simulink library "reelInOut"  (R2018a)
settings: Solver=VariableStepAuto  StartTime=0.0  StopTime=10.0  RelTol=1e-3
undefined symbols (not defined in the file or in its folder): ctrl, plant
libraries: controllerComponents x9, simulink x6
settings Model: Creator=mitch  LastModifiedBy=mitch

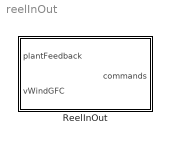
== system reelInOut ==
  ReelInOut : Subsystem  VariantControl=variantOCKReelInOut

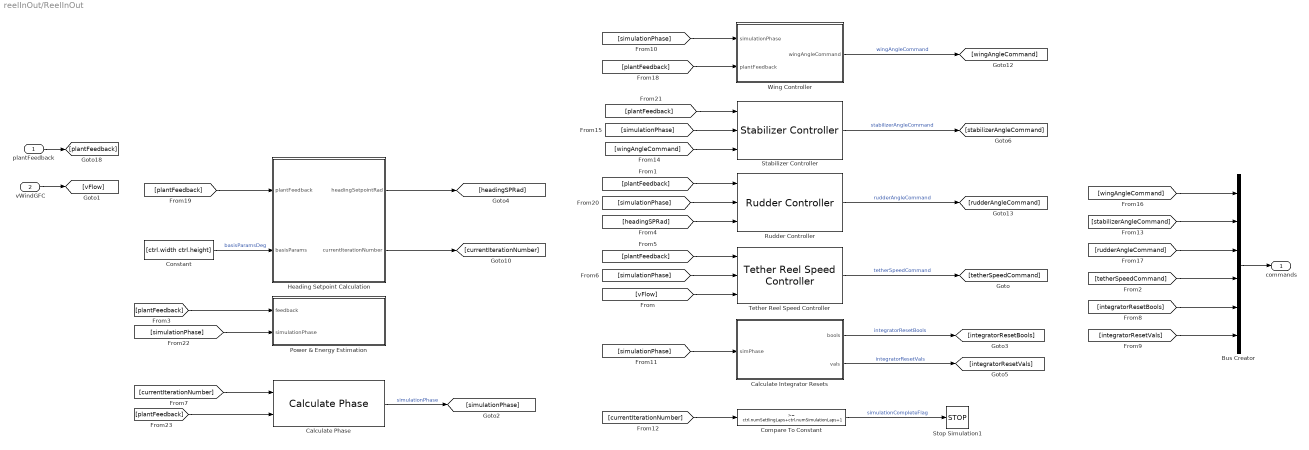
== system reelInOut/ReelInOut ==
  plantFeedback : Inport  OutDataTypeStr=Bus: busPlantFeedback
  vWindGFC : Inport  Port=2
  Bus Creator : BusCreator  Inputs=6  OutDataTypeStr=Bus: busControllerOutput
  Calculate Integrator Resets : Subsystem
  Calculate Phase : controllerComponents/Calculate Phase
  Compare To Constant : simulink/Logic and Bit Operations/Compare To Constant  relop=>=  const=ctrl.numSettlingLaps+ctrl.numSimulationLaps+1  OutDataTypeStr=boolean
  Constant : Constant  Value=[ctrl.width ctrl.height]
  Heading Setpoint Calculation : Subsystem  VariantControl=variantPureCarrotFollowing
  Power & Energy Estimation : Subsystem
  Rudder Controller : controllerComponents/Rudder Controller
  Stabilizer Controller : controllerComponents/Stabilizer Controller
  Stop Simulation1 : Stop
  Tether Reel Speed Controller : controllerComponents/Tether Reel Speed Controller
  Wing Controller : Subsystem
  commands : Outport  OutDataTypeStr=Bus: busControllerOutput
  wires:
  [plantFeedback] -> Calculate Phase/2
  [simulationPhase] -> Power & Energy Estimation/2(simulationPhase)
  [wingAngleCommand] -> Stabilizer Controller/3
  [plantFeedback] -> Stabilizer Controller/1
  [simulationPhase] -> Stabilizer Controller/2
  [simulationPhase] -> Rudder Controller/2
  [headingSPRad] -> Rudder Controller/3
  [plantFeedback] -> Rudder Controller/1
  [stabilizerAngleCommand] -> Bus Creator/2
  Stabilizer Controller/1 -> [stabilizerAngleCommand]  "stabilizerAngleCommand"
  [wingAngleCommand] -> Bus Creator/1
  [rudderAngleCommand] -> Bus Creator/3
  [tetherSpeedCommand] -> Bus Creator/4
  [integratorResetBools] -> Bus Creator/5
  [integratorResetVals] -> Bus Creator/6
  [simulationPhase] -> Tether Reel Speed Controller/2
  [plantFeedback] -> Tether Reel Speed Controller/1
  [vFlow] -> Tether Reel Speed Controller/3
  Calculate Integrator Resets/2(vals) -> [integratorResetVals]  "integratorResetVals"
  Calculate Integrator Resets/1(bools) -> [integratorResetBools]  "integratorResetBools"
  [simulationPhase] -> Calculate Integrator Resets/1(simPhase)
  [simulationPhase] -> Wing Controller/1(simulationPhase)
  Wing Controller/1(wingAngleCommand) -> [wingAngleCommand]  "wingAngleCommand"
  [plantFeedback] -> Wing Controller/2(plantFeedback)
  Calculate Phase/1 -> [simulationPhase]  "simulationPhase"
  [currentIterationNumber] -> Calculate Phase/1
  [plantFeedback] -> Power & Energy Estimation/1(feedback)
  Tether Reel Speed Controller/1 -> [tetherSpeedCommand]  "tetherSpeedCommand"
  Rudder Controller/1 -> [rudderAngleCommand]  "rudderAngleCommand"
  Heading Setpoint Calculation/1(headingSetpointRad) -> [headingSPRad]
  Heading Setpoint Calculation/2(currentIterationNumber) -> [currentIterationNumber]
  Compare To Constant/1 -> Stop Simulation1/1  "simulationCompleteFlag"
  [currentIterationNumber] -> Compare To Constant/1
  Bus Creator/1 -> commands/1
  vWindGFC/1 -> [vFlow]
  plantFeedback/1 -> [plantFeedback]
  Constant/1 -> Heading Setpoint Calculation/2(basisParams)  "basisParamsDeg"
  [plantFeedback] -> Heading Setpoint Calculation/1(plantFeedback)

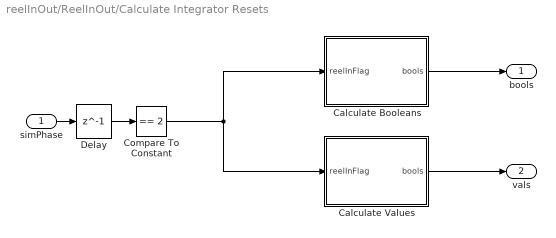
== system reelInOut/ReelInOut/Calculate Integrator Resets ==
  simPhase : Inport
  Calculate Booleans : Subsystem
  Calculate Values : Subsystem
  Compare To Constant : simulink/Logic and Bit Operations/Compare To Constant  relop===  const=2  OutDataTypeStr=boolean
  Delay : Delay  DelayLength=1  InitialCondition=0
  bools : Outport
  vals : Outport  Port=2
  wires:
  Delay/1 -> Compare To Constant/1
  Compare To Constant/1 -> Calculate Values/1(reelInFlag), Calculate Booleans/1(reelInFlag)
  Calculate Values/1(bools) -> vals/1
  Calculate Booleans/1(bools) -> bools/1
  simPhase/1 -> Delay/1

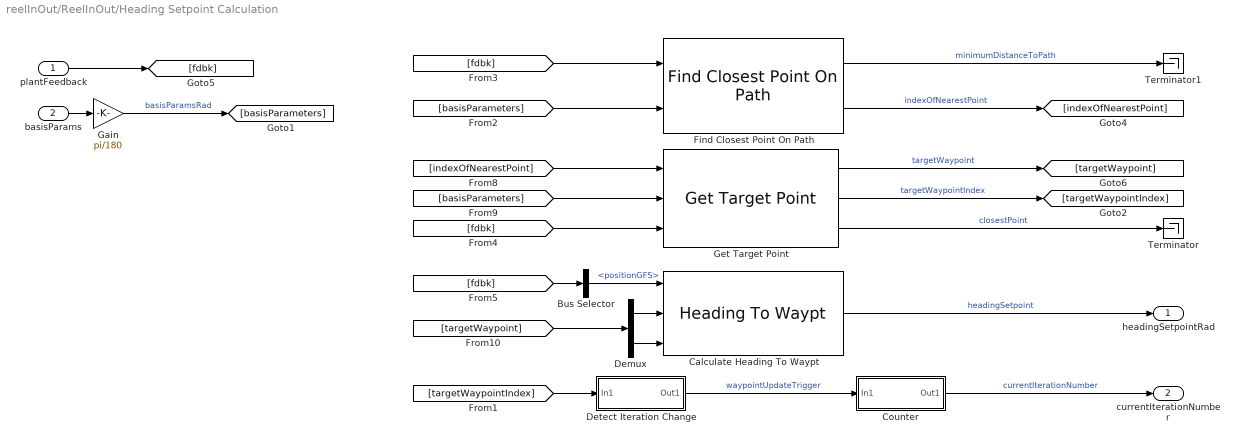
== system reelInOut/ReelInOut/Heading Setpoint Calculation ==
  plantFeedback : Inport  OutDataTypeStr=Bus: busPlantFeedback
  basisParams : Inport  Port=2
  Bus Selector : BusSelector  OutputSignals=positionGFS
  Calculate Heading To Waypt : controllerComponents/Heading To Waypt
  Counter : Subsystem
  Demux : Demux  Outputs=2
  Detect Iteration Change : Subsystem
  Find Closest Point On Path : controllerComponents/Find Closest Point On Path
  Gain : Gain  Gain=pi/180
  Get Target Point : controllerComponents/Get Target Point
  Terminator : Terminator
  Terminator1 : Terminator
  headingSetpointRad : Outport
  currentIterationNumber : Outport  Port=2
  wires:
  Gain/1 -> [basisParameters]  "basisParamsRad"
  Bus Selector/1 -> Calculate Heading To Waypt/1  "<positionGFS>"
  [fdbk] -> Bus Selector/1
  basisParams/1 -> Gain/1
  [fdbk] -> Get Target Point/3
  [fdbk] -> Find Closest Point On Path/1
  [basisParameters] -> Find Closest Point On Path/2
  Demux/1 -> Calculate Heading To Waypt/2
  Demux/2 -> Calculate Heading To Waypt/3
  Find Closest Point On Path/1 -> Terminator1/1  "minimumDistanceToPath"
  Find Closest Point On Path/2 -> [indexOfNearestPoint]  "indexOfNearestPoint"
  [indexOfNearestPoint] -> Get Target Point/1
  [basisParameters] -> Get Target Point/2
  Get Target Point/1 -> [targetWaypoint]  "targetWaypoint"
  [targetWaypoint] -> Demux/1
  Calculate Heading To Waypt/1 -> headingSetpointRad/1  "headingSetpoint"
  [targetWaypointIndex] -> Detect Iteration Change/1(In1)
  Counter/1(Out1) -> currentIterationNumber/1  "currentIterationNumber"
  Detect Iteration Change/1(Out1) -> Counter/1(In1)  "waypointUpdateTrigger"
  Get Target Point/2 -> [targetWaypointIndex]  "targetWaypointIndex"
  plantFeedback/1 -> [fdbk]
  Get Target Point/3 -> Terminator/1  "closestPoint"

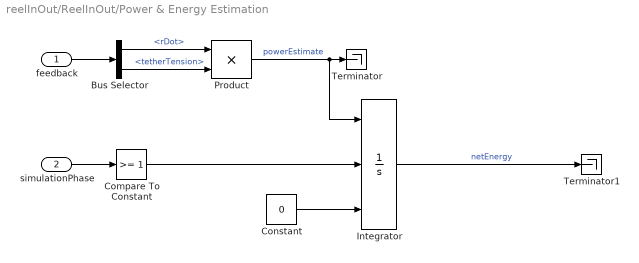
== system reelInOut/ReelInOut/Power & Energy Estimation ==
  feedback : Inport
  simulationPhase : Inport  Port=2
  Bus Selector : BusSelector  OutputSignals=rDot,tetherTension
  Compare To Constant : simulink/Logic and Bit Operations/Compare To Constant  relop=>=  const=1  OutDataTypeStr=boolean
  Constant : Constant  Value=0
  Integrator : Integrator  ExternalReset=rising  InitialConditionSource=external
  Product : Product
  Terminator : Terminator
  Terminator1 : Terminator
  wires:
  Constant/1 -> Integrator/3
  Compare To Constant/1 -> Integrator/2
  simulationPhase/1 -> Compare To Constant/1
  Integrator/1 -> Terminator1/1  "netEnergy"
  Bus Selector/2 -> Product/2  "<tetherTension>"
  Bus Selector/1 -> Product/1  "<rDot>"
  feedback/1 -> Bus Selector/1
  Product/1 -> Terminator/1, Integrator/1  "powerEstimate"

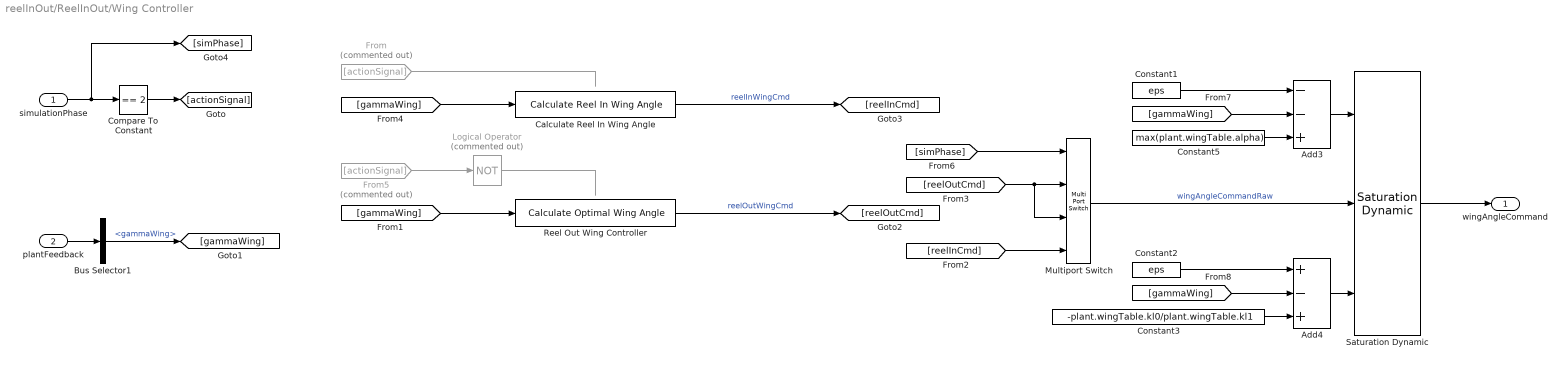
== system reelInOut/ReelInOut/Wing Controller ==
  simulationPhase : Inport
  plantFeedback : Inport  Port=2
  Add3 : Sum  Inputs=--+
  Add4 : Sum  Inputs=+-+
  Bus Selector1 : BusSelector  OutputSignals=gammaWing
  Calculate Reel In Wing Angle : controllerComponents/Calculate Reel In Wing Angle
  Compare To Constant : simulink/Logic and Bit Operations/Compare To Constant  relop===  const=2  OutDataTypeStr=boolean
  Constant1 : Constant  Value=eps
  Constant2 : Constant  Value=eps
  Constant3 : Constant  Value=-plant.wingTable.kl0/plant.wingTable.kl1
  Constant5 : Constant  Value=max(plant.wingTable.alpha)
  From : From  Commented=on  GotoTag=actionSignal
  From5 : From  Commented=on  GotoTag=actionSignal
  Logical Operator : Logic  Commented=on  Operator=NOT  AllPortsSameDT=off  OutDataTypeStr=boolean
  Multiport Switch : MultiPortSwitch  DataPortOrder=Zero-based contiguous  zeroidx=on
  Reel Out Wing Controller : controllerComponents/Calculate Optimal Wing Angle
  Saturation Dynamic : simulink/Discontinuities/Saturation Dynamic  OutMin=[]  OutMax=[]  OutDataTypeStr=Inherit: Same as second input  OutDataType=fixdt(1, 16)  OutScaling=2^-10  DoSatur=off
  wingAngleCommand : Outport
  wires:
  [reelInCmd] -> Multiport Switch/4
  [reelOutCmd] -> Multiport Switch/2, Multiport Switch/3
  [simPhase] -> Multiport Switch/1
  Multiport Switch/1 -> Saturation Dynamic/2  "wingAngleCommandRaw"
  Constant2/1 -> Add4/1
  [gammaWing] -> Add4/2
  Constant3/1 -> Add4/3
  [gammaWing] -> Add3/2
  Constant1/1 -> Add3/1
  Constant5/1 -> Add3/3
  From5/1 -> Logical Operator/1
  From/1 -> ?
  Compare To Constant/1 -> [actionSignal]
  Logical Operator/1 -> ?
  [gammaWing] -> Calculate Reel In Wing Angle/1
  Calculate Reel In Wing Angle/1 -> [reelInCmd]  "reelInWingCmd"
  Reel Out Wing Controller/1 -> [reelOutCmd]  "reelOutWingCmd"
  [gammaWing] -> Reel Out Wing Controller/1
  Bus Selector1/1 -> [gammaWing]  "<gammaWing>"
  Saturation Dynamic/1 -> wingAngleCommand/1
  Add3/1 -> Saturation Dynamic/1
  Add4/1 -> Saturation Dynamic/3
  simulationPhase/1 -> Compare To Constant/1, [simPhase]
  plantFeedback/1 -> Bus Selector1/1

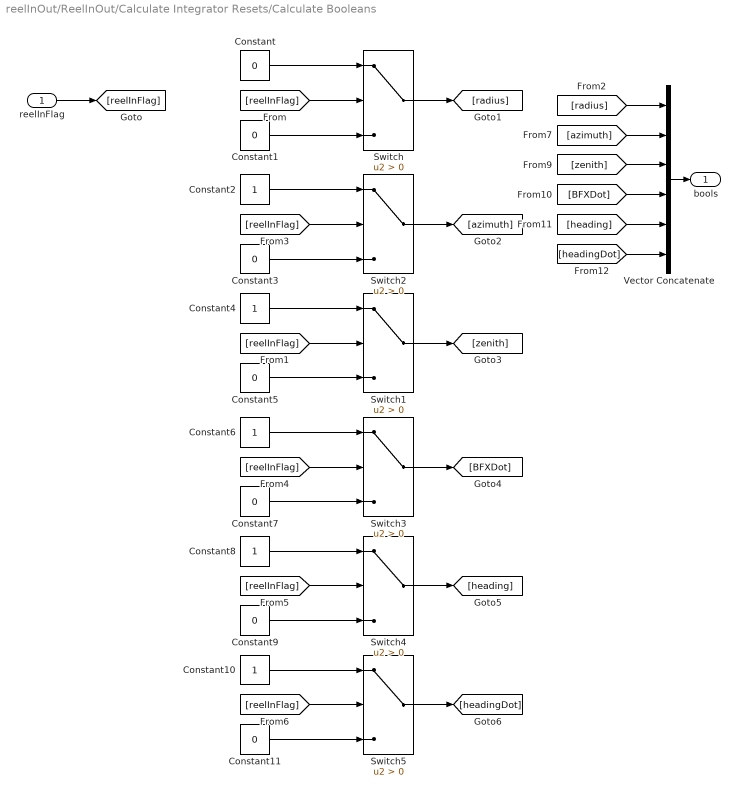
== system reelInOut/ReelInOut/Calculate Integrator Resets/Calculate Booleans ==
  reelInFlag : Inport
  Constant{,1,3,5,7,9,11} (7 alike) : Constant  Value=0  OutDataTypeStr=boolean
  Constant{2,4,6,8,10} (5 alike) : Constant  OutDataTypeStr=boolean
  Switch{,1..5} (6 alike) : Switch  Criteria=u2 > Threshold
  Vector Concatenate : Concatenate  NumInputs=6
  bools : Outport
  wires:
  reelInFlag/1 -> [reelInFlag]
  [headingDot] -> Vector Concatenate/6
  [reelInFlag] -> Switch2/2
  Switch2/1 -> [azimuth]
  Constant3/1 -> Switch2/3
  Constant2/1 -> Switch2/1
  [heading] -> Vector Concatenate/5
  [zenith] -> Vector Concatenate/3
  [azimuth] -> Vector Concatenate/2
  Vector Concatenate/1 -> bools/1
  Switch3/1 -> [BFXDot]
  Constant6/1 -> Switch3/1
  [reelInFlag] -> Switch3/2
  Constant7/1 -> Switch3/3
  Constant1/1 -> Switch/3
  Switch/1 -> [radius]
  [BFXDot] -> Vector Concatenate/4
  Constant/1 -> Switch/1
  Constant11/1 -> Switch5/3
  Constant10/1 -> Switch5/1
  Switch5/1 -> [headingDot]
  [reelInFlag] -> Switch5/2
  [radius] -> Vector Concatenate/1
  Switch1/1 -> [zenith]
  [reelInFlag] -> Switch/2
  [reelInFlag] -> Switch1/2
  Constant4/1 -> Switch1/1
  Constant5/1 -> Switch1/3
  [reelInFlag] -> Switch4/2
  Constant9/1 -> Switch4/3
  Switch4/1 -> [heading]
  Constant8/1 -> Switch4/1

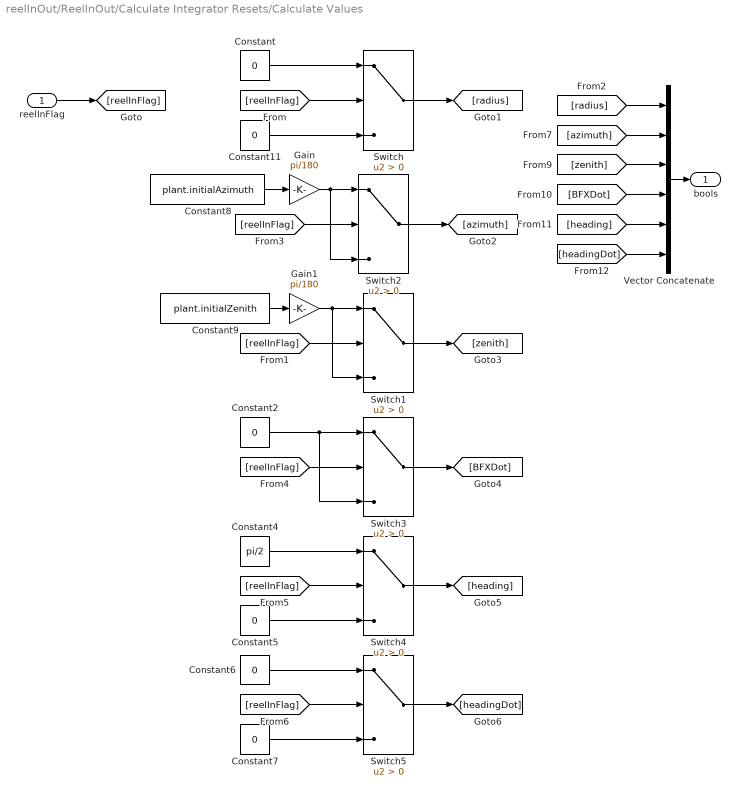
== system reelInOut/ReelInOut/Calculate Integrator Resets/Calculate Values ==
  reelInFlag : Inport
  Constant{,2,5..7,11} (6 alike) : Constant  Value=0  OutDataTypeStr=double
  Constant4 : Constant  Value=pi/2  OutDataTypeStr=double
  Constant8 : Constant  Value=plant.initialAzimuth  OutDataTypeStr=double
  Constant9 : Constant  Value=plant.initialZenith  OutDataTypeStr=double
  Gain : Gain  Gain=pi/180
  Gain1 : Gain  Gain=pi/180
  Switch{,1..5} (6 alike) : Switch  Criteria=u2 > Threshold
  Vector Concatenate : Concatenate  NumInputs=6
  bools : Outport
  wires:
  reelInFlag/1 -> [reelInFlag]
  [headingDot] -> Vector Concatenate/6
  [reelInFlag] -> Switch2/2
  Switch2/1 -> [azimuth]
  Gain/1 -> Switch2/1, Switch2/3
  Constant8/1 -> Gain/1
  [heading] -> Vector Concatenate/5
  [zenith] -> Vector Concatenate/3
  [azimuth] -> Vector Concatenate/2
  Vector Concatenate/1 -> bools/1
  Switch3/1 -> [BFXDot]
  [reelInFlag] -> Switch3/2
  Constant2/1 -> Switch3/1, Switch3/3
  Constant11/1 -> Switch/3
  Switch/1 -> [radius]
  [BFXDot] -> Vector Concatenate/4
  Constant/1 -> Switch/1
  Constant7/1 -> Switch5/3
  Constant6/1 -> Switch5/1
  Switch5/1 -> [headingDot]
  [reelInFlag] -> Switch5/2
  [radius] -> Vector Concatenate/1
  Switch1/1 -> [zenith]
  [reelInFlag] -> Switch/2
  [reelInFlag] -> Switch1/2
  Constant9/1 -> Gain1/1
  Gain1/1 -> Switch1/1, Switch1/3
  [reelInFlag] -> Switch4/2
  Constant5/1 -> Switch4/3
  Switch4/1 -> [heading]
  Constant4/1 -> Switch4/1

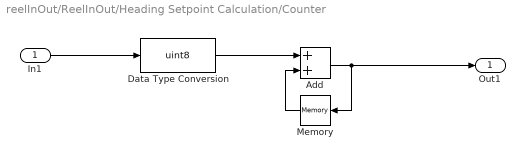
== system reelInOut/ReelInOut/Heading Setpoint Calculation/Counter ==
  In1 : Inport
  Add : Sum
  Data Type Conversion : DataTypeConversion  OutDataTypeStr=uint8
  Memory : Memory  InitialCondition=1
  Out1 : Outport  OutDataTypeStr=double
  wires:
  Add/1 -> Out1/1, Memory/1
  Memory/1 -> Add/2
  In1/1 -> Data Type Conversion/1
  Data Type Conversion/1 -> Add/1

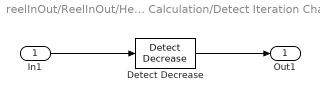
== system reelInOut/ReelInOut/Heading Setpoint Calculation/Detect Iteration Change ==
  In1 : Inport
  Detect Decrease : simulink/Logic and Bit Operations/Detect Decrease  vinit=0.0  OutDataTypeStr=boolean
  Out1 : Outport
  wires:
  In1/1 -> Detect Decrease/1
  Detect Decrease/1 -> Out1/1
